simulink model "LATC_Test_Calc4"  (R2021b)
settings: Solver=FixedStepDiscrete  StartTime=49.3316  StopTime=94.3708  FixedStep=0.01  RelTol=1e-3
values from neighbouring files (symbols this model uses):
  P_Global_CharSpd_ms : value not decoded    [PubParsGlobal.sldd]
  P_Global_SteeringAngleRatio : value not decoded    [PubParsGlobal.sldd]
  P_Global_WheelBase_m : value not decoded    [PubParsGlobal.sldd]
  P_LCS_Current_Offset_Test_SW = 0.0    [LATC.sldd]
  P_LCS_Current_Offset_Test_Value = 0.0    [LATC.sldd]
  P_LCS_Curvature_bp : value not decoded    [LATC.sldd]
  P_LCS_CycleTime = 0.4 0.4 0.4 0.4 0.4 0.4 0.4 0.4 0.4 0.6 0.6 0.6 0.6 0.6 0.6 0.6 0.4 0.4 0.4 0.4 0.4 0.4 0.4 0.4 0.4 0.6 0.6 0.6 0.6 0.6 0.6 0.6 0.4 0.4 0.4 0.4 0.4 0.4 0.4 0.4 0.4 0.6 0.6 0.6 0.6 0.6 0.6 0.6 0.4 0.4 0.4 0.4 0.4 0.4 0.4 0.4 0.4 0.6 0.6 0.6 0.6 0.6 0.6 0.6 0.4 0.4 0.4 0.4 0.4 0.4 0.4 0.4 0.4 0.6 0.6 0.6 0.6 0.6 0.6 0.6 0.4 0.4 0.4 0.4 0.4 0.4 0.4 0.4 0.4 0.6 0.6 0.6 0.6 0.6 0.6 0.6 0.4 0.4 0.4 0.4    [LATC.sldd]
  P_LCS_ESS_AngleSlope_Limit = 2.9    [LATC.sldd]    (also in LCS_v05.sldd)
  P_LCS_LATC_CurOffsetVehicleSpdLimitValue_degs = 7.0    [LATC.sldd]
  P_LCS_LATC_Du_Max = 20.0    [LATC.sldd]
  P_LCS_LATC_ELKAngleSlope_ratio : value not decoded    [LATC.sldd]
  P_LCS_LATC_ELKMaxLatAcc_ms2 : value not decoded    [LATC.sldd]
  P_LCS_LATC_ESSAngleSlope_ratio : value not decoded    [LATC.sldd]
  P_LCS_LATC_ESSMaxLatAcc_ms2 : value not decoded    [LATC.sldd]
  P_LCS_LATC_LCAngleSlope_ratio : value not decoded    [LATC.sldd]
  P_LCS_LATC_LCCancleMaxLatAcc_ms2 : value not decoded    [LATC.sldd]
  P_LCS_LATC_LCEcoAngleSlope_ratio : value not decoded    [LATC.sldd]
  P_LCS_LATC_LCEcoMaxLatAcc_ms2 : value not decoded    [LATC.sldd]
  P_LCS_LATC_LCKAngleSlope_ratio : value not decoded    [LATC.sldd]
  P_LCS_LATC_LCKIEAngleSlope_ratio : value not decoded    [LATC.sldd]
  P_LCS_LATC_LCKIEMaxLatAcc_ms2 : value not decoded    [LATC.sldd]
  P_LCS_LATC_LCKMaxLatAcc_ms2 : value not decoded    [LATC.sldd]
  P_LCS_LATC_LCNormalAngleSlope_ratio : value not decoded    [LATC.sldd]
  P_LCS_LATC_LCNormalMaxLatAcc_ms2 : value not decoded    [LATC.sldd]
  P_LCS_LATC_LCSportAngleSlope_ratio : value not decoded    [LATC.sldd]
  P_LCS_LATC_LCSportMaxLatAcc_ms2 : value not decoded    [LATC.sldd]
  P_LCS_LATC_LKAAngleSlope_ratio : value not decoded    [LATC.sldd]
  P_LCS_LATC_LKAMaxLatAcc_ms2 : value not decoded    [LATC.sldd]
  P_LCS_LATC_MatrixQ1_st = 0.8 0.8 1.2 1.4 1.4 1.4 2.0 2.2 2.2 2.2 2.2 2.2 2.2 2.2 2.2 2.2 0.8 0.8 1.2 1.4 1.4 1.4 2.0 2.2 2.2 2.2 2.2 2.2 2.2 2.2 2.2 2.2 0.8 0.8 1.2 1.4 1.4 1.4 2.0 2.2 2.2 2.2 2.2 2.2 2.2 2.2 2.2 2.2 0.8 0.8 1.2 1.4 1.4 1.4 2.0 2.2 2.2 2.2 2.2 2.2 2.2 2.2 2.2 2.2 0.8 0.8 1.2 1.4 1.4 1.4 2.0 2.2 2.2 2.2 2.2 2.2 2.2 2.2 2.2 2.2 0.8 0.8 1.2 1.4 1.4 1.4 2.0 2.2 2.2 2.2 2.2 2.2 2.2 2.2 2.2 2.2 0.8 0.8 1.2 1.4    [LATC.sldd]
  P_LCS_LATC_MatrixQ3_st = 20.0 20.0 20.0 20.0 20.0 15.0 15.0 15.0 15.0 15.0 15.0 15.0 15.0 13.0 13.0 13.0 20.0 20.0 20.0 20.0 20.0 15.0 15.0 15.0 15.0 15.0 15.0 15.0 15.0 13.0 13.0 13.0 20.0 20.0 20.0 20.0 20.0 15.0 15.0 15.0 15.0 15.0 15.0 15.0 15.0 13.0 13.0 13.0 20.0 20.0 20.0 20.0 20.0 15.0 15.0 15.0 15.0 15.0 15.0 15.0 15.0 13.0 13.0 13.0 20.0 20.0 20.0 20.0 20.0 15.0 15.0 15.0 15.0 15.0 15.0 15.0 15.0 13.0 13.0 13.0    [LATC.sldd]
  P_LCS_LATC_MatrixR_st = 10.0 10.0 10.0 10.0 10.0 10.0 10.0 15.0 15.0 15.0 15.0 15.0 15.0 15.0 15.0 15.0 10.0 10.0 10.0 10.0 10.0 10.0 10.0 15.0 15.0 15.0 15.0 15.0 15.0 15.0 15.0 15.0 10.0 10.0 10.0 10.0 10.0 10.0 10.0 15.0 15.0 15.0 15.0 15.0 15.0 15.0 15.0 15.0 10.0 10.0 10.0 10.0 10.0 10.0 10.0 15.0 15.0 15.0 15.0 15.0 15.0 15.0 15.0 15.0 10.0 10.0 10.0 10.0 10.0 10.0 10.0 15.0 15.0 15.0 15.0 15.0 15.0 15.0 15.0 15.0    [LATC.sldd]
  P_LCS_LATC_Max_LatAcc = 4.0    [LATC.sldd]
  P_LCS_LATC_Max_Phi = 15.0    [LATC.sldd]
  P_LCS_LATC_Max_y = 0.5    [LATC.sldd]
  P_LCS_LATC_MPC_SW = 0.0    [LATC.sldd]
  P_LCS_LATC_PreView_SW = 1.0    [LATC.sldd]
  P_LCS_LATC_SoftConstWeight = 1.0    [LATC.sldd]
  P_LCS_LATC_StateActivAngleSlopeLimit_ratio : value not decoded    [LATC.sldd]
  P_LCS_LATC_StateActiveFlg_TabX_st : value not decoded    [LATC.sldd]
  P_LCS_LATC_StateActiveHoldTime_TabY_st : value not decoded    [LATC.sldd]
  P_LCS_LATC_StateHoldTime_st = 250.0    [LATC.sldd]
  P_LCS_LATC_TarAngleFliterWindowSize = 5.0    [LATC.sldd]
  P_LCS_LATC_TarAngleLP_Time = 0.02    [LATC.sldd]
  P_LCS_LATC_U_Max = 90.0    [LATC.sldd]
  P_LCS_LCK_AngleSlope_Limit = 1.4    [LATC.sldd]
  P_LCS_LineVaildSW = 0.0    [LATC.sldd]
  P_LCS_Lookahead_Distance : value not decoded    [LATC.sldd]
  P_LCS_Lookahead_DistanceFac : value not decoded    [LATC.sldd]
  P_LCS_PLAN_CurvePreView_s = 0.3    [LATC.sldd]
  P_LCS_PLAN_CurvePreview_TabX_m : value not decoded    [LATC.sldd]
  P_LCS_PLAN_CurvePreViewFilterTime_s = 0.1    [LATC.sldd]
  P_LCS_PLAN_ELKAyDtLimit_Tab_ms3 = 1.0 1.0 1.0 1.0 1.0 1.0 1.0 1.0 1.0 1.0 1.0 1.0 1.0 1.0 1.0 1.0 1.0 1.0 1.0 1.0 1.0 1.0 1.0 1.0 1.0 1.0 1.0 1.0 1.0 1.0 1.0 1.0 1.0 1.0 1.0 1.0 1.0 1.0 1.0 1.0 1.0 1.0 1.0 1.0 1.0 1.0 1.0 1.0 1.0 1.0 1.0 1.0 1.0 1.0 1.0 1.0 1.0 1.0 1.0 1.0 1.0 1.0 1.0 1.0 1.0 1.0 1.0 1.0 1.0 1.0 1.0 1.0 1.0 1.0 1.0 1.0 1.0 1.0 1.0 1.0 1.0 1.0 1.0 1.0 1.0 1.0 1.0 1.0 1.0 1.0 1.0 1.0 1.0 1.0 1.0 1.0 1.0 1.0 1.0 1.0    [LATC.sldd]
  P_LCS_PLAN_ESSAyDtLimit_Tab_ms3 = 1.0 1.0 1.0 1.0 1.0 1.0 1.0 1.0 1.0 1.0 1.0 1.0 1.0 1.0 1.0 1.0 1.0 1.0 1.0 1.0 1.0 1.0 1.0 1.0 1.0 1.0 1.0 1.0 1.0 1.0 1.0 1.0 1.0 1.0 1.0 1.0 1.0 1.0 1.0 1.0 1.0 1.0 1.0 1.0 1.0 1.0 1.0 1.0 1.0 1.0 1.0 1.0 1.0 1.0 1.0 1.0 1.0 1.0 1.0 1.0 1.0 1.0 1.0 1.0 1.0 1.0 1.0 1.0 1.0 1.0 1.0 1.0 1.0 1.0 1.0 1.0 1.0 1.0 1.0 1.0 1.0 1.0 1.0 1.0 1.0 1.0 1.0 1.0 1.0 1.0 1.0 1.0 1.0 1.0 1.0 1.0 1.0 1.0 1.0 1.0    [LATC.sldd]
  P_LCS_PLAN_LCCancleAyDtLimit_Tab_ms3 = 1.0 1.0 1.0 1.0 1.0 1.0 1.0 1.0 1.0 1.0 1.0 1.0 1.0 1.0 1.0 1.0 1.0 1.0 1.0 1.0 1.0 1.0 1.0 1.0 1.0 1.0 1.0 1.0 1.0 1.0 1.0 1.0 1.0 1.0 1.0 1.0 1.0 1.0 1.0 1.0 1.0 1.0 1.0 1.0 1.0 1.0 1.0 1.0 1.0 1.0 1.0 1.0 1.0 1.0 1.0 1.0 1.0 1.0 1.0 1.0 1.0 1.0 1.0 1.0 1.0 1.0 1.0 1.0 1.0 1.0 1.0 1.0 1.0 1.0 1.0 1.0 1.0 1.0 1.0 1.0 1.0 1.0 1.0 1.0 1.0 1.0 1.0 1.0 1.0 1.0 1.0 1.0 1.0 1.0 1.0 1.0 1.0 1.0 1.0 1.0    [LATC.sldd]
  P_LCS_PLAN_LCEcoAyDtLimit_Tab_ms3 = 1.0 1.0 1.0 1.0 1.0 1.0 1.0 1.0 1.0 1.0 1.0 1.0 1.0 1.0 1.0 1.0 1.0 1.0 1.0 1.0 1.0 1.0 1.0 1.0 1.0 1.0 1.0 1.0 1.0 1.0 1.0 1.0 1.0 1.0 1.0 1.0 1.0 1.0 1.0 1.0 1.0 1.0 1.0 1.0 1.0 1.0 1.0 1.0 1.0 1.0 1.0 1.0 1.0 1.0 1.0 1.0 1.0 1.0 1.0 1.0 1.0 1.0 1.0 1.0 1.0 1.0 1.0 1.0 1.0 1.0 1.0 1.0 1.0 1.0 1.0 1.0 1.0 1.0 1.0 1.0 1.0 1.0 1.0 1.0 1.0 1.0 1.0 1.0 1.0 1.0 1.0 1.0 1.0 1.0 1.0 1.0 1.0 1.0 1.0 1.0    [LATC.sldd]
  P_LCS_PLAN_LCKAyDtLimit_Tab_ms3 = 1.5 1.5 1.5 1.5 1.5 1.5 1.5 1.5 1.5 1.5 1.5 1.5 1.5 1.5 1.5 1.5 1.5 1.5 1.5 1.5 1.5 1.5 1.5 1.5 1.5 1.5 1.5 1.5 1.5 1.5 1.5 1.5 1.5 1.5 1.5 1.5 1.5 1.5 1.5 1.5 1.5 1.5 1.5 1.5 1.5 1.5 1.5 1.5 1.5 1.5 1.5 1.5 1.5 1.5 1.5 1.5 1.5 1.5 1.5 1.5 1.5 1.5 1.5 1.5 1.5 1.5 1.5 1.5 1.5 1.5 1.5 1.5 1.5 1.5 1.5 1.5 1.5 1.5 1.5 1.5 1.5 1.5 1.5 1.5 1.5 1.5 1.5 1.5 1.5 1.5 1.5 1.5 1.5 1.5 1.5 1.5 1.5 1.5 1.5 1.5    [LATC.sldd]
  P_LCS_PLAN_LCKIEAyDtLimit_Tab_ms3 = 1.0 1.0 1.0 1.0 1.0 1.0 1.0 1.0 1.0 1.0 1.0 1.0 1.0 1.0 1.0 1.0 1.0 1.0 1.0 1.0 1.0 1.0 1.0 1.0 1.0 1.0 1.0 1.0 1.0 1.0 1.0 1.0 1.0 1.0 1.0 1.0 1.0 1.0 1.0 1.0 1.0 1.0 1.0 1.0 1.0 1.0 1.0 1.0 1.0 1.0 1.0 1.0 1.0 1.0 1.0 1.0 1.0 1.0 1.0 1.0 1.0 1.0 1.0 1.0 1.0 1.0 1.0 1.0 1.0 1.0 1.0 1.0 1.0 1.0 1.0 1.0 1.0 1.0 1.0 1.0 1.0 1.0 1.0 1.0 1.0 1.0 1.0 1.0 1.0 1.0 1.0 1.0 1.0 1.0 1.0 1.0 1.0 1.0 1.0 1.0    [LATC.sldd]
  P_LCS_PLAN_LCNormalAyDtLimit_Tab_ms3 = 1.0 1.0 1.0 1.0 1.0 1.0 1.0 1.0 1.0 1.0 1.0 1.0 1.0 1.0 1.0 1.0 1.0 1.0 1.0 1.0 1.0 1.0 1.0 1.0 1.0 1.0 1.0 1.0 1.0 1.0 1.0 1.0 1.0 1.0 1.0 1.0 1.0 1.0 1.0 1.0 1.0 1.0 1.0 1.0 1.0 1.0 1.0 1.0 1.0 1.0 1.0 1.0 1.0 1.0 1.0 1.0 1.0 1.0 1.0 1.0 1.0 1.0 1.0 1.0 1.0 1.0 1.0 1.0 1.0 1.0 1.0 1.0 1.0 1.0 1.0 1.0 1.0 1.0 1.0 1.0 1.0 1.0 1.0 1.0 1.0 1.0 1.0 1.0 1.0 1.0 1.0 1.0 1.0 1.0 1.0 1.0 1.0 1.0 1.0 1.0    [LATC.sldd]
  P_LCS_PLAN_LCSportAyDtLimit_Tab_ms3 = 1.0 1.0 1.0 1.0 1.0 1.0 1.0 1.0 1.0 1.0 1.0 1.0 1.0 1.0 1.0 1.0 1.0 1.0 1.0 1.0 1.0 1.0 1.0 1.0 1.0 1.0 1.0 1.0 1.0 1.0 1.0 1.0 1.0 1.0 1.0 1.0 1.0 1.0 1.0 1.0 1.0 1.0 1.0 1.0 1.0 1.0 1.0 1.0 1.0 1.0 1.0 1.0 1.0 1.0 1.0 1.0 1.0 1.0 1.0 1.0 1.0 1.0 1.0 1.0 1.0 1.0 1.0 1.0 1.0 1.0 1.0 1.0 1.0 1.0 1.0 1.0 1.0 1.0 1.0 1.0 1.0 1.0 1.0 1.0 1.0 1.0 1.0 1.0 1.0 1.0 1.0 1.0 1.0 1.0 1.0 1.0 1.0 1.0 1.0 1.0    [LATC.sldd]
  P_LCS_PLAN_LKAAyDtLimit_Tab_ms3 = 1.0 1.0 1.0 1.0 1.0 1.0 1.0 1.0 1.0 1.0 1.0 1.0 1.0 1.0 1.0 1.0 1.0 1.0 1.0 1.0 1.0 1.0 1.0 1.0 1.0 1.0 1.0 1.0 1.0 1.0 1.0 1.0 1.0 1.0 1.0 1.0 1.0 1.0 1.0 1.0 1.0 1.0 1.0 1.0 1.0 1.0 1.0 1.0 1.0 1.0 1.0 1.0 1.0 1.0 1.0 1.0 1.0 1.0 1.0 1.0 1.0 1.0 1.0 1.0 1.0 1.0 1.0 1.0 1.0 1.0 1.0 1.0 1.0 1.0 1.0 1.0 1.0 1.0 1.0 1.0 1.0 1.0 1.0 1.0 1.0 1.0 1.0 1.0 1.0 1.0 1.0 1.0 1.0 1.0 1.0 1.0 1.0 1.0 1.0 1.0    [LATC.sldd]
  P_LCS_PLAN_MinPlanDis_m : value not decoded    [LATC.sldd]
  P_LCS_PLAN_PreCurMinDisFac_ratio : value not decoded    [LATC.sldd]
  P_LCS_PLAN_PreDisCurve_TabX_m : value not decoded    [LATC.sldd]
  P_LCS_PLAN_StateActiv_AyDtLimit_ms3 : value not decoded    [LATC.sldd]
  P_LCS_PLAN_VehicleSpd_TabX_kph : value not decoded    [LATC.sldd]
  P_LCS_PLAN_VehicleSpd_TabY_Kph : value not decoded    [LATC.sldd]
  P_LCS_VehicleSpd_TabX_Kph : value not decoded    [LATC.sldd]
libraries: simulink x3, dspbuff3 x2
(part 3 of 4)

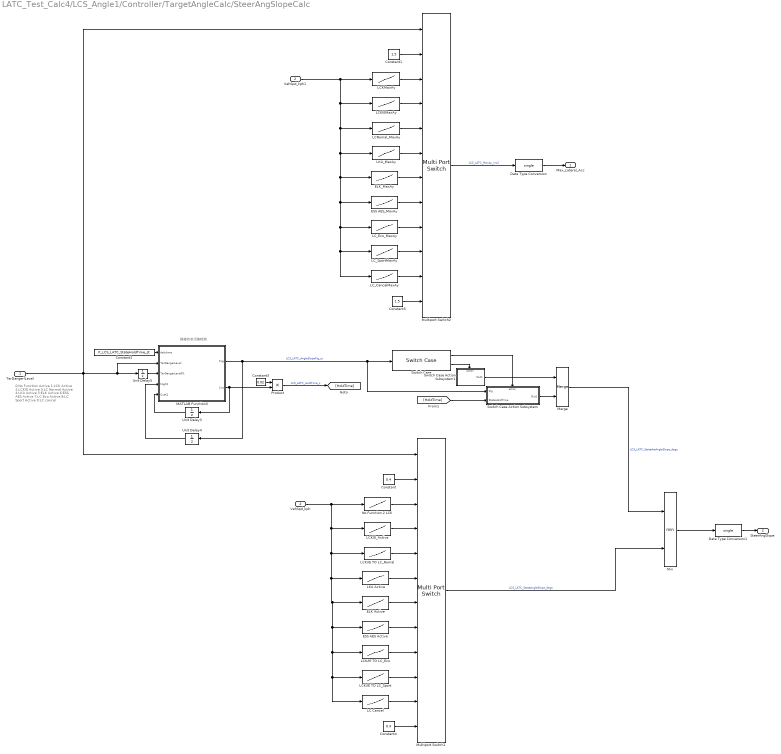
== system LATC_Test_Calc4/LCS_Angle1/Controller/TargetAngleCalc/SteerAngSlopeCalc ==
  note: 0:No Function Active
      | 1:LCK Active
      | 2:LCKIE Active
      | 3:LC Normal Active
      | 4:LKA Active
      | 5:ELK Active
      | 6:ESS AES Active
      | 7:LC Eco Active
      | 8:LC Sport Active
      | 9:LC cancel
  note: 换道状态切换检测
  TarDangerlLevel : Inport
  VehSpd_kph : Inport  Port=2
  Constant : Constant  Value=0.4  OutDataTypeStr=single
  Constant1 : Constant  Value=1.5  OutDataTypeStr=single
  Constant2 : Constant  Value=P_LCS_LATC_StateHoldTime_st  OutDataTypeStr=uint16
  Constant3 : Constant  Value=0.02
  Constant4 : Constant  Value=0.4  OutDataTypeStr=single
  Constant5 : Constant  Value=1.5  OutDataTypeStr=single
  Data Type Conversion : DataTypeConversion  OutDataTypeStr=single
  Data Type Conversion1 : DataTypeConversion  OutDataTypeStr=single
  ELK Active : Lookup_n-D  NumberOfTableDimensions=1  BreakpointsForDimension1=P_LCS_VehicleSpd_TabX_Kph  Table=P_LCS_LATC_ELKAngleSlope_ratio  ExtrapMethod=Clip  InternalRulePriority=Speed  RndMeth=Simplest  InputSameDT=on
  ELK_MaxAy : Lookup_n-D  NumberOfTableDimensions=1  BreakpointsForDimension1=P_LCS_VehicleSpd_TabX_Kph  Table=P_LCS_LATC_ELKMaxLatAcc_ms2  ExtrapMethod=Clip  InternalRulePriority=Speed  RndMeth=Simplest  InputSameDT=on
  ESS AES Active : Lookup_n-D  NumberOfTableDimensions=1  BreakpointsForDimension1=P_LCS_VehicleSpd_TabX_Kph  Table=P_LCS_LATC_ESSAngleSlope_ratio  ExtrapMethod=Clip  InternalRulePriority=Speed  RndMeth=Simplest  InputSameDT=on
  ESS AES_MaxAy : Lookup_n-D  NumberOfTableDimensions=1  BreakpointsForDimension1=P_LCS_VehicleSpd_TabX_Kph  Table=P_LCS_LATC_ESSMaxLatAcc_ms2  ExtrapMethod=Clip  InternalRulePriority=Speed  RndMeth=Simplest  InputSameDT=on
  LC Cancel : Lookup_n-D  NumberOfTableDimensions=1  BreakpointsForDimension1=P_LCS_VehicleSpd_TabX_Kph  Table=P_LCS_LATC_LCAngleSlope_ratio  ExtrapMethod=Clip  InternalRulePriority=Speed  RndMeth=Simplest  InputSameDT=on
  LCK/IE TO LC_Eco : Lookup_n-D  NumberOfTableDimensions=1  BreakpointsForDimension1=P_LCS_VehicleSpd_TabX_Kph  Table=P_LCS_LATC_LCEcoAngleSlope_ratio  ExtrapMethod=Clip  InternalRulePriority=Speed  RndMeth=Simplest  InputSameDT=on
  LCK/IE TO LC_Nomal : Lookup_n-D  NumberOfTableDimensions=1  BreakpointsForDimension1=P_LCS_VehicleSpd_TabX_Kph  Table=P_LCS_LATC_LCNormalAngleSlope_ratio  ExtrapMethod=Clip  InternalRulePriority=Speed  RndMeth=Simplest  InputSameDT=on
  LCK/IE TO LC_Sport : Lookup_n-D  NumberOfTableDimensions=1  BreakpointsForDimension1=P_LCS_VehicleSpd_TabX_Kph  Table=P_LCS_LATC_LCSportAngleSlope_ratio  ExtrapMethod=Clip  InternalRulePriority=Speed  RndMeth=Simplest  InputSameDT=on
  LCKIEMaxAy : Lookup_n-D  NumberOfTableDimensions=1  BreakpointsForDimension1=P_LCS_VehicleSpd_TabX_Kph  Table=P_LCS_LATC_LCKIEMaxLatAcc_ms2  ExtrapMethod=Clip  InternalRulePriority=Speed  RndMeth=Simplest  InputSameDT=on
  LCKIE_Active : Lookup_n-D  NumberOfTableDimensions=1  BreakpointsForDimension1=P_LCS_VehicleSpd_TabX_Kph  Table=P_LCS_LATC_LCKIEAngleSlope_ratio  ExtrapMethod=Clip  InternalRulePriority=Speed  RndMeth=Simplest  InputSameDT=on
  LCKMaxAy : Lookup_n-D  NumberOfTableDimensions=1  BreakpointsForDimension1=P_LCS_VehicleSpd_TabX_Kph  Table=P_LCS_LATC_LCKMaxLatAcc_ms2  ExtrapMethod=Clip  InternalRulePriority=Speed  RndMeth=Simplest  InputSameDT=on
  LCNomal_MaxAy : Lookup_n-D  NumberOfTableDimensions=1  BreakpointsForDimension1=P_LCS_VehicleSpd_TabX_Kph  Table=P_LCS_LATC_LCNormalMaxLatAcc_ms2  ExtrapMethod=Clip  InternalRulePriority=Speed  RndMeth=Simplest  InputSameDT=on
  LC_CancelMaxAy : Lookup_n-D  NumberOfTableDimensions=1  BreakpointsForDimension1=P_LCS_VehicleSpd_TabX_Kph  Table=P_LCS_LATC_LCCancleMaxLatAcc_ms2  ExtrapMethod=Clip  InternalRulePriority=Speed  RndMeth=Simplest  InputSameDT=on
  LC_Eco_MaxAy : Lookup_n-D  NumberOfTableDimensions=1  BreakpointsForDimension1=P_LCS_VehicleSpd_TabX_Kph  Table=P_LCS_LATC_LCEcoMaxLatAcc_ms2  ExtrapMethod=Clip  InternalRulePriority=Speed  RndMeth=Simplest  InputSameDT=on
  LC_SportMaxAy : Lookup_n-D  NumberOfTableDimensions=1  BreakpointsForDimension1=P_LCS_VehicleSpd_TabX_Kph  Table=P_LCS_LATC_LCSportMaxLatAcc_ms2  ExtrapMethod=Clip  InternalRulePriority=Speed  RndMeth=Simplest  InputSameDT=on
  LKA Active : Lookup_n-D  NumberOfTableDimensions=1  BreakpointsForDimension1=P_LCS_VehicleSpd_TabX_Kph  Table=P_LCS_LATC_LKAAngleSlope_ratio  ExtrapMethod=Clip  InternalRulePriority=Speed  RndMeth=Simplest  InputSameDT=on
  LKA_MaxAy : Lookup_n-D  NumberOfTableDimensions=1  BreakpointsForDimension1=P_LCS_VehicleSpd_TabX_Kph  Table=P_LCS_LATC_LKAMaxLatAcc_ms2  ExtrapMethod=Clip  InternalRulePriority=Speed  RndMeth=Simplest  InputSameDT=on
  MATLAB Function3 : MATLAB Function  TreatAsAtomicUnit=on
  Merge : Merge
  Min : MinMax  Inputs=2
  Multiport Switch1 : MultiPortSwitch  DataPortOrder=Zero-based contiguous  Inputs=11  zeroidx=on
  Multiport Switch2 : MultiPortSwitch  DataPortOrder=Zero-based contiguous  Inputs=11  zeroidx=on
  No Function 2 LCK : Lookup_n-D  NumberOfTableDimensions=1  BreakpointsForDimension1=P_LCS_VehicleSpd_TabX_Kph  Table=P_LCS_LATC_LCKAngleSlope_ratio  ExtrapMethod=Clip  InternalRulePriority=Speed  RndMeth=Simplest  InputSameDT=on
  Product : Product
  Switch Case : SwitchCase  CaseConditions={[1,2,3,4,5]}
  Switch Case Action Subsystem : Subsystem  TreatAsAtomicUnit=on
  Switch Case Action Subsystem1 : Subsystem  TreatAsAtomicUnit=on
  Unit Delay3 : UnitDelay  SampleTime=-1  HasFrameUpgradeWarning=on
  Unit Delay4 : UnitDelay  SampleTime=-1  HasFrameUpgradeWarning=on
  Unit Delay5 : UnitDelay  SampleTime=-1  HasFrameUpgradeWarning=on
  VehSpd_kph1 : InportShadow  Port=2
  Max_Lateral_Acc : Outport  OutDataTypeStr=single
  SteerAngSlope : Outport  Port=2  OutDataTypeStr=single
  wires:
  TarDangerlLevel/1 -> Multiport Switch1/1, Multiport Switch2/1, Unit Delay5/1, MATLAB Function3/2(TarDangerLevel)
  Merge/1 -> Min/1  "LCS_LATC_StateActAngleSlope_degs"
  Switch Case Action Subsystem1/1(Out1) -> Merge/1
  Switch Case Action Subsystem/1(Out1) -> Merge/2
  [HoldTime] -> Switch Case Action Subsystem/2(StateHoldTime)
  Switch Case/2 -> Switch Case Action Subsystem1/Action
  Switch Case/1 -> Switch Case Action Subsystem/Action
  LCK/IE TO LC_Nomal/1 -> Multiport Switch1/5
  Min/1 -> Data Type Conversion1/1
  Product/1 -> [HoldTime]  "LCS_LATC_HoldTime_s"
  Constant3/1 -> Product/1
  Constant4/1 -> Multiport Switch1/12
  LKA Active/1 -> Multiport Switch1/6
  No Function 2 LCK/1 -> Multiport Switch1/3
  Multiport Switch1/1 -> Min/2  "LCS_LATC_StateAngleSlope_degs"
  Constant2/1 -> MATLAB Function3/1(delytime)
  MATLAB Function3/1(FLg) -> Unit Delay4/1, Switch Case Action Subsystem/1(Flg), Switch Case/1  "LCS_LATC_AngleSlopeFlg_st"
  MATLAB Function3/2(Cnt) -> Unit Delay3/1, Product/2
  Constant/1 -> Multiport Switch1/2
  Unit Delay4/1 -> MATLAB Function3/4(FLgK1)
  Unit Delay3/1 -> MATLAB Function3/5(CntK1)
  LCKIE_Active/1 -> Multiport Switch1/4
  ELK Active/1 -> Multiport Switch1/7
  VehSpd_kph/1 -> No Function 2 LCK/1, LCK/IE TO LC_Nomal/1, LC Cancel/1, LCK/IE TO LC_Sport/1, LCK/IE TO LC_Eco/1, ESS AES Active/1, ELK Active/1, LKA Active/1, LCKIE_Active/1
  Unit Delay5/1 -> MATLAB Function3/3(TarDangerLevelK1)
  ESS AES Active/1 -> Multiport Switch1/8
  LCK/IE TO LC_Eco/1 -> Multiport Switch1/9
  LCK/IE TO LC_Sport/1 -> Multiport Switch1/10
  LC Cancel/1 -> Multiport Switch1/11
  Multiport Switch2/1 -> Data Type Conversion/1  "LCS_LATC_MaxAy_ms2"
  Constant1/1 -> Multiport Switch2/2
  Constant5/1 -> Multiport Switch2/12
  LC_CancelMaxAy/1 -> Multiport Switch2/11
  LC_SportMaxAy/1 -> Multiport Switch2/10
  LC_Eco_MaxAy/1 -> Multiport Switch2/9
  ESS AES_MaxAy/1 -> Multiport Switch2/8
  VehSpd_kph1/1 -> LCKIEMaxAy/1, LKA_MaxAy/1, ELK_MaxAy/1, ESS AES_MaxAy/1, LC_Eco_MaxAy/1, LC_SportMaxAy/1, LC_CancelMaxAy/1, LCNomal_MaxAy/1, LCKMaxAy/1
  ELK_MaxAy/1 -> Multiport Switch2/7
  LCKIEMaxAy/1 -> Multiport Switch2/4
  LCKMaxAy/1 -> Multiport Switch2/3
  LKA_MaxAy/1 -> Multiport Switch2/6
  LCNomal_MaxAy/1 -> Multiport Switch2/5
  Data Type Conversion/1 -> Max_Lateral_Acc/1
  Data Type Conversion1/1 -> SteerAngSlope/1

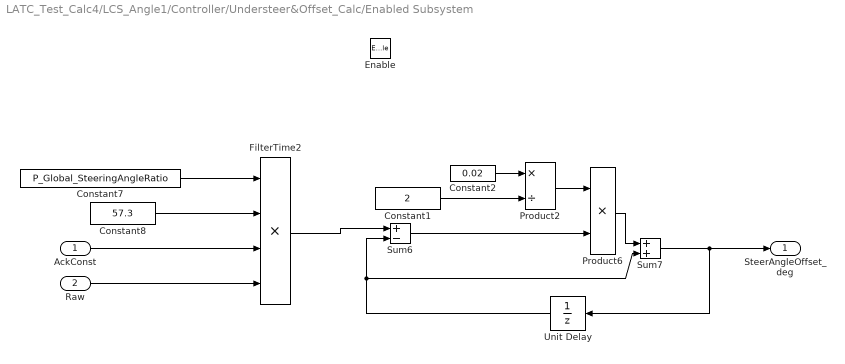
== system LATC_Test_Calc4/LCS_Angle1/Controller/Understeer&Offset_Calc/Enabled Subsystem ==
  AckConst : Inport
  Raw : Inport  Port=2
  Enable : EnablePort
  Constant1 : Constant  Value=2  OutDataTypeStr=single
  Constant2 : Constant  Value=0.02  OutDataTypeStr=single
  Constant7 : Constant  Value=P_Global_SteeringAngleRatio
  Constant8 : Constant  Value=57.3  OutDataTypeStr=single
  FilterTime2 : Product  Inputs=4  RndMeth=Zero
  Product2 : Product  Inputs=*/  RndMeth=Zero
  Product6 : Product  RndMeth=Zero
  Sum6 : Sum  Inputs=+-
  Sum7 : Sum
  Unit Delay : UnitDelay  SampleTime=-1  HasFrameUpgradeWarning=on
  SteerAngleOffset_deg : Outport
  wires:
  Constant1/1 -> Product2/2
  FilterTime2/1 -> Sum6/1
  Raw/1 -> FilterTime2/4
  AckConst/1 -> FilterTime2/3
  Constant8/1 -> FilterTime2/2
  Constant7/1 -> FilterTime2/1
  Product6/1 -> Sum7/1
  Product2/1 -> Product6/1
  Sum6/1 -> Product6/2
  Constant2/1 -> Product2/1
  Unit Delay/1 -> Sum7/2, Sum6/2
  Sum7/1 -> Unit Delay/1, SteerAngleOffset_deg/1

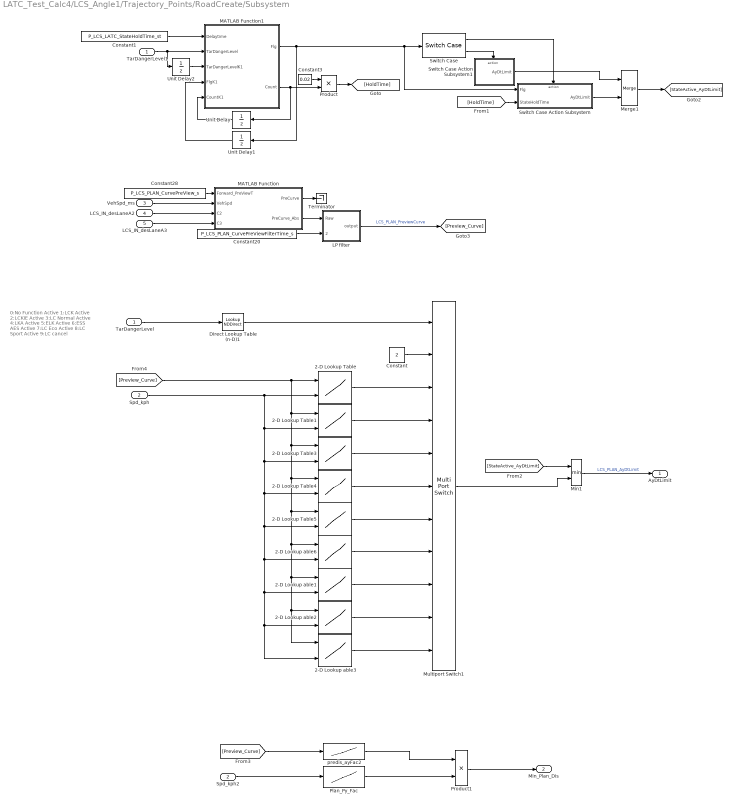
== system LATC_Test_Calc4/LCS_Angle1/Trajectory_Points/RoadCreate/Subsystem ==
  note: 0:No Function Active
      | 1:LCK Active
      | 2:LCKIE Active
      | 3:LC Normal Active
      | 4:LKA Active
      | 5:ELK Active
      | 6:ESS AES Active
      | 7:LC Eco Active
      | 8:LC Sport Active
      | 9:LC cancel
  TarDangerLevel : Inport
  Spd_kph : Inport  Port=2
  VehSpd_ms : Inport  Port=3
  LCS_IN_desLaneA2 : Inport  Port=4
  LCS_IN_desLaneA3 : Inport  Port=5
  2-D Lookup Table : Lookup_n-D  BreakpointsForDimension1=P_LCS_PLAN_PreDisCurve_TabX_m  BreakpointsForDimension2=P_LCS_PLAN_VehicleSpd_TabY_Kph  Table=P_LCS_PLAN_LCKAyDtLimit_Tab_ms3  InternalRulePriority=Speed  RndMeth=Simplest  InputSameDT=on
      settings: InputPortMap=u0,u1
  2-D Lookup Table1 : Lookup_n-D  BreakpointsForDimension1=P_LCS_PLAN_PreDisCurve_TabX_m  BreakpointsForDimension2=P_LCS_PLAN_VehicleSpd_TabY_Kph  Table=P_LCS_PLAN_LCKIEAyDtLimit_Tab_ms3  InternalRulePriority=Speed  RndMeth=Simplest  InputSameDT=on
      settings: InputPortMap=u0,u1
  2-D Lookup Table3 : Lookup_n-D  BreakpointsForDimension1=P_LCS_PLAN_PreDisCurve_TabX_m  BreakpointsForDimension2=P_LCS_PLAN_VehicleSpd_TabY_Kph  Table=P_LCS_PLAN_LCNormalAyDtLimit_Tab_ms3  InternalRulePriority=Speed  RndMeth=Simplest  InputSameDT=on
      settings: InputPortMap=u0,u1
  2-D Lookup Table4 : Lookup_n-D  BreakpointsForDimension1=P_LCS_PLAN_PreDisCurve_TabX_m  BreakpointsForDimension2=P_LCS_PLAN_VehicleSpd_TabY_Kph  Table=P_LCS_PLAN_LKAAyDtLimit_Tab_ms3  InternalRulePriority=Speed  RndMeth=Simplest  InputSameDT=on
      settings: InputPortMap=u0,u1
  2-D Lookup Table5 : Lookup_n-D  BreakpointsForDimension1=P_LCS_PLAN_PreDisCurve_TabX_m  BreakpointsForDimension2=P_LCS_PLAN_VehicleSpd_TabY_Kph  Table=P_LCS_PLAN_ELKAyDtLimit_Tab_ms3  InternalRulePriority=Speed  RndMeth=Simplest  InputSameDT=on
      settings: InputPortMap=u0,u1
  2-D Lookup able1 : Lookup_n-D  BreakpointsForDimension1=P_LCS_PLAN_PreDisCurve_TabX_m  BreakpointsForDimension2=P_LCS_PLAN_VehicleSpd_TabY_Kph  Table=P_LCS_PLAN_LCEcoAyDtLimit_Tab_ms3  InternalRulePriority=Speed  RndMeth=Simplest  InputSameDT=on
      settings: InputPortMap=u0,u1
  2-D Lookup able2 : Lookup_n-D  BreakpointsForDimension1=P_LCS_PLAN_PreDisCurve_TabX_m  BreakpointsForDimension2=P_LCS_PLAN_VehicleSpd_TabY_Kph  Table=P_LCS_PLAN_LCSportAyDtLimit_Tab_ms3  InternalRulePriority=Speed  RndMeth=Simplest  InputSameDT=on
      settings: InputPortMap=u0,u1
  2-D Lookup able3 : Lookup_n-D  BreakpointsForDimension1=P_LCS_PLAN_PreDisCurve_TabX_m  BreakpointsForDimension2=P_LCS_PLAN_VehicleSpd_TabY_Kph  Table=P_LCS_PLAN_LCCancleAyDtLimit_Tab_ms3  InternalRulePriority=Speed  RndMeth=Simplest  InputSameDT=on
      settings: InputPortMap=u0,u1
  2-D Lookup able6 : Lookup_n-D  BreakpointsForDimension1=P_LCS_PLAN_PreDisCurve_TabX_m  BreakpointsForDimension2=P_LCS_PLAN_VehicleSpd_TabY_Kph  Table=P_LCS_PLAN_ESSAyDtLimit_Tab_ms3  InternalRulePriority=Speed  RndMeth=Simplest  InputSameDT=on
      settings: InputPortMap=u0,u1
  Constant : Constant  Value=2  OutDataTypeStr=single
  Constant1 : Constant  Value=P_LCS_LATC_StateHoldTime_st  OutDataTypeStr=uint16
  Constant20 : Constant  Value=P_LCS_PLAN_CurvePreViewFilterTime_s  OutDataTypeStr=single
  Constant28 : Constant  Value=P_LCS_PLAN_CurvePreView_s  OutDataTypeStr=single
  Constant3 : Constant  Value=0.02
  Direct Lookup Table (n-D)1 : LookupNDDirect  NumberOfTableDimensions=1  Table=[0 1 2 3 4 5 6 7 8 9]  TableDataTypeStr=uint8
  LP filter : Subsystem
  MATLAB Function : MATLAB Function  TreatAsAtomicUnit=on
  MATLAB Function1 : MATLAB Function  TreatAsAtomicUnit=on
  Merge1 : Merge
  Min1 : MinMax  Inputs=2
  Multiport Switch1 : MultiPortSwitch  DataPortOrder=Zero-based contiguous  Inputs=10  zeroidx=on
  Plan_Py_Fac : Lookup_n-D  NumberOfTableDimensions=1  BreakpointsForDimension1=P_LCS_PLAN_VehicleSpd_TabX_kph  Table=P_LCS_PLAN_MinPlanDis_m  ExtrapMethod=Clip  UseLastTableValue=on  InternalRulePriority=Speed  RndMeth=Simplest  InputSameDT=on
  Product : Product
  Product1 : Product
  Spd_kph2 : InportShadow  Port=2
  Switch Case : SwitchCase  CaseConditions={[1]}
  Switch Case Action Subsystem : Subsystem  TreatAsAtomicUnit=on
  Switch Case Action Subsystem1 : Subsystem  TreatAsAtomicUnit=on
  TarDangerLevel1 : InportShadow
  Terminator : Terminator
  Unit Delay : UnitDelay  SampleTime=-1  HasFrameUpgradeWarning=on
  Unit Delay1 : UnitDelay  SampleTime=-1  HasFrameUpgradeWarning=on
  Unit Delay2 : UnitDelay  SampleTime=-1  HasFrameUpgradeWarning=on
  predis_ayFac2 : Lookup_n-D  NumberOfTableDimensions=1  BreakpointsForDimension1=P_LCS_PLAN_CurvePreview_TabX_m  Table=P_LCS_PLAN_PreCurMinDisFac_ratio  ExtrapMethod=Clip  UseLastTableValue=on  InternalRulePriority=Speed  RndMeth=Simplest  InputSameDT=on
  AyDtLimit : Outport  OutDataTypeStr=single
  Min_Plan_Dis : Outport  Port=2  OutDataTypeStr=single
  wires:
  2-D Lookup Table/1 -> Multiport Switch1/3
  Multiport Switch1/1 -> Min1/2
  [StateActive_AyDtLimit] -> Min1/1
  Merge1/1 -> [StateActive_AyDtLimit]
  Switch Case Action Subsystem1/1(AyDtLimit) -> Merge1/1
  Switch Case Action Subsystem/1(AyDtLimit) -> Merge1/2
  Product/1 -> [HoldTime]
  [HoldTime] -> Switch Case Action Subsystem/2(StateHoldTime)
  Constant3/1 -> Product/1
  Switch Case/2 -> Switch Case Action Subsystem1/Action
  MATLAB Function1/2(Count) -> Unit Delay/1, Product/2
  Switch Case/1 -> Switch Case Action Subsystem/Action
  MATLAB Function1/1(Flg) -> Switch Case/1, Switch Case Action Subsystem/1(Flg), Unit Delay1/1
  Constant1/1 -> MATLAB Function1/1(Delaytime)
  Unit Delay2/1 -> MATLAB Function1/3(TarDangerLevelK1)
  TarDangerLevel1/1 -> MATLAB Function1/2(TarDangerLevel), Unit Delay2/1
  Unit Delay1/1 -> MATLAB Function1/4(FlgK1)
  Unit Delay/1 -> MATLAB Function1/5(CountK1)
  2-D Lookup Table5/1 -> Multiport Switch1/7
  2-D Lookup Table3/1 -> Multiport Switch1/5
  2-D Lookup Table1/1 -> Multiport Switch1/4
  Constant/1 -> Multiport Switch1/2
  Constant28/1 -> MATLAB Function/1(Forward_PreViewT)
  LP filter/1(output) -> [Preview_Curve]  "LCS_PLAN_PreviewCurve"
  Constant20/1 -> LP filter/2(TorqFilterTime)
  LCS_IN_desLaneA3/1 -> MATLAB Function/4(C3)
  LCS_IN_desLaneA2/1 -> MATLAB Function/3(C2)
  VehSpd_ms/1 -> MATLAB Function/2(VehSpd)
  Min1/1 -> AyDtLimit/1  "LCS_PLAN_AyDtLimit"
  TarDangerLevel/1 -> Direct Lookup Table (n-D)1/1
  Direct Lookup Table (n-D)1/1 -> Multiport Switch1/1
  Plan_Py_Fac/1 -> Product1/2
  Spd_kph2/1 -> Plan_Py_Fac/1
  [Preview_Curve] -> predis_ayFac2/1
  Product1/1 -> Min_Plan_Dis/1
  predis_ayFac2/1 -> Product1/1
  MATLAB Function/2(PreCurve_Abs) -> LP filter/1(Raw)
  MATLAB Function/1(PreCurve) -> Terminator/1
  [Preview_Curve] -> 2-D Lookup able3/1, 2-D Lookup able2/1, 2-D Lookup able1/1, 2-D Lookup able6/1, 2-D Lookup Table5/1, 2-D Lookup Table4/1, 2-D Lookup Table3/1, 2-D Lookup Table1/1, 2-D Lookup Table/1
  Spd_kph/1 -> 2-D Lookup Table/2, 2-D Lookup Table1/2, 2-D Lookup Table3/2, 2-D Lookup Table4/2, 2-D Lookup able3/2, 2-D Lookup able2/2, 2-D Lookup able1/2, 2-D Lookup able6/2, 2-D Lookup Table5/2
  2-D Lookup Table4/1 -> Multiport Switch1/6
  2-D Lookup able6/1 -> Multiport Switch1/8
  2-D Lookup able1/1 -> Multiport Switch1/9
  2-D Lookup able2/1 -> Multiport Switch1/10
  2-D Lookup able3/1 -> Multiport Switch1/11

== system LATC_Test_Calc4/LCS_Angle1/Controller/TargetAngleCalc/MedianLowPass_Filter/LP ==
  Raw : Inport
  Constant1 : Constant  Value=P_LCS_LATC_TarAngleLP_Time  OutDataTypeStr=single
  Constant3 : Constant  Value=0.02  OutDataTypeStr=single
  Product7 : Product  Inputs=*/  RndMeth=Zero
  Product8 : Product  RndMeth=Zero
  Sum14 : Sum
  Sum9 : Sum  Inputs=+-
  Unit Delay : UnitDelay  SampleTime=-1  HasFrameUpgradeWarning=on
  Out : Outport
  wires:
  Constant1/1 -> Product7/2
  Constant3/1 -> Product7/1
  Sum9/1 -> Product8/2
  Sum14/1 -> Out/1, Unit Delay/1
  Unit Delay/1 -> Sum14/2, Sum9/2
  Raw/1 -> Sum9/1
  Product8/1 -> Sum14/1
  Product7/1 -> Product8/1

== system LATC_Test_Calc4/LCS_Angle1/Controller/TargetAngleCalc/MedianLowPass_Filter/Median_Filter ==
  In : Inport
  Add : Sum  Inputs=+-
  Constant : Constant  Value=2  OutDataTypeStr=single
  Constant11 : Constant  Value=P_LCS_LATC_TarAngleFliterWindowSize  OutDataTypeStr=single
  Delay Line : dspbuff3/Delay Line  siz=P_LCS_LATC_TarAngleFliterWindowSize  ic=0  directfeed=off  enable_output=off  hold_output=off  OutputFrames=off
      settings: SourceProductBaseCode=DS
  Divide1 : Product  Inputs=*/
  Max of Elements1 : MinMax  Function=max
  MinMax2 : MinMax
  Minus1 : Sum  Inputs=--+
  Sum of Elements1 : Sum  Inputs=+
  Out : Outport
  wires:
  Max of Elements1/1 -> Minus1/2
  Divide1/1 -> Out/1
  Minus1/1 -> Divide1/1
  In/1 -> Delay Line/1
  MinMax2/1 -> Minus1/1
  Sum of Elements1/1 -> Minus1/3
  Delay Line/1 -> Max of Elements1/1, MinMax2/1, Sum of Elements1/1
  Constant11/1 -> Add/1
  Add/1 -> Divide1/2
  Constant/1 -> Add/2

== system LATC_Test_Calc4/LCS_Angle1/Controller/TargetAngleCalc/MedianLowPass_Filter1/LP ==
  Raw : Inport
  Constant1 : Constant  Value=0.02  OutDataTypeStr=single
  Constant3 : Constant  Value=0.02  OutDataTypeStr=single
  Product7 : Product  Inputs=*/  RndMeth=Zero
  Product8 : Product  RndMeth=Zero
  Sum14 : Sum
  Sum9 : Sum  Inputs=+-
  Unit Delay : UnitDelay  SampleTime=-1  HasFrameUpgradeWarning=on
  Out : Outport
  wires:
  Constant1/1 -> Product7/2
  Constant3/1 -> Product7/1
  Sum9/1 -> Product8/2
  Sum14/1 -> Out/1, Unit Delay/1
  Unit Delay/1 -> Sum14/2, Sum9/2
  Raw/1 -> Sum9/1
  Product8/1 -> Sum14/1
  Product7/1 -> Product8/1

== system LATC_Test_Calc4/LCS_Angle1/Controller/TargetAngleCalc/MedianLowPass_Filter1/Median_Filter ==
  In : Inport
  Add : Sum  Inputs=+-
  Constant : Constant  Value=2  OutDataTypeStr=single
  Constant11 : Constant  Value=P_LCS_LATC_TarAngleFliterWindowSize  OutDataTypeStr=single
  Delay Line : dspbuff3/Delay Line  siz=P_LCS_LATC_TarAngleFliterWindowSize  ic=0  directfeed=off  enable_output=off  hold_output=off  OutputFrames=off
      settings: SourceProductBaseCode=DS
  Divide1 : Product  Inputs=*/
  Max of Elements1 : MinMax  Function=max
  MinMax2 : MinMax
  Minus1 : Sum  Inputs=--+
  Sum of Elements1 : Sum  Inputs=+
  Out : Outport
  wires:
  Max of Elements1/1 -> Minus1/2
  Divide1/1 -> Out/1
  Minus1/1 -> Divide1/1
  In/1 -> Delay Line/1
  MinMax2/1 -> Minus1/1
  Sum of Elements1/1 -> Minus1/3
  Delay Line/1 -> Max of Elements1/1, MinMax2/1, Sum of Elements1/1
  Constant11/1 -> Add/1
  Add/1 -> Divide1/2
  Constant/1 -> Add/2

== system LATC_Test_Calc4/LCS_Angle1/Controller/TargetAngleCalc/SteerAngSlopeCalc/Switch Case Action Subsystem ==
  Flg : Inport
  StateHoldTime : Inport  Port=2
  Action Port : ActionPort  ActionPortLabel=case [ 1 2 3 4 5 ]:
  LC_start_slope : Lookup_n-D  BreakpointsForDimension1=P_LCS_LATC_StateActiveFlg_TabX_st  BreakpointsForDimension2=P_LCS_LATC_StateActiveHoldTime_TabY_st  Table=P_LCS_LATC_StateActivAngleSlopeLimit_ratio  ExtrapMethod=Clip  UseLastTableValue=on  InternalRulePriority=Speed  OutDataTypeStr=single  RndMeth=Simplest
      settings: InputPortMap=u0,u1
  Out1 : Outport
  wires:
  StateHoldTime/1 -> LC_start_slope/2
  LC_start_slope/1 -> Out1/1
  Flg/1 -> LC_start_slope/1

== system LATC_Test_Calc4/LCS_Angle1/Controller/TargetAngleCalc/SteerAngSlopeCalc/Switch Case Action Subsystem1 ==
  Action Port : ActionPort  ActionPortLabel=default:
  Constant : Constant  Value=100  OutDataTypeStr=single
  Out1 : Outport
  wires:
  Constant/1 -> Out1/1

== system LATC_Test_Calc4/LCS_Angle1/Trajectory_Points/RoadCreate/Subsystem/LP filter ==
  Raw : Inport
  TorqFilterTime : Inport  Port=2
  Product1 : Product  RndMeth=Zero
  Product4 : Product  Inputs=*/  RndMeth=Zero
  Sum4 : Sum  Inputs=+-
  Sum5 : Sum
  Unit Delay : UnitDelay  SampleTime=-1  HasFrameUpgradeWarning=on
  Weight/N3 : Constant  Value=0.02  OutDataTypeStr=single
  output : Outport
  wires:
  TorqFilterTime/1 -> Product4/2
  Product4/1 -> Product1/1
  Weight/N3/1 -> Product4/1
  Raw/1 -> Sum4/1
  Product1/1 -> Sum5/1
  Sum4/1 -> Product1/2
  Unit Delay/1 -> Sum4/2, Sum5/2
  Sum5/1 -> Unit Delay/1, output/1

== system LATC_Test_Calc4/LCS_Angle1/Trajectory_Points/RoadCreate/Subsystem/Switch Case Action Subsystem ==
  Flg : Inport
  StateHoldTime : Inport  Port=2
  Action Port : ActionPort  ActionPortLabel=case [ 1 ]:
  ActiveAyDtLimit_TBL : Lookup_n-D  BreakpointsForDimension1=P_LCS_LATC_StateActiveFlg_TabX_st  BreakpointsForDimension2=P_LCS_LATC_StateActiveHoldTime_TabY_st  Table=P_LCS_PLAN_StateActiv_AyDtLimit_ms3  ExtrapMethod=Clip  UseLastTableValue=on  InternalRulePriority=Speed  OutDataTypeStr=single  RndMeth=Simplest
      settings: InputPortMap=u0,u1
  AyDtLimit : Outport
  wires:
  ActiveAyDtLimit_TBL/1 -> AyDtLimit/1
  Flg/1 -> ActiveAyDtLimit_TBL/1
  StateHoldTime/1 -> ActiveAyDtLimit_TBL/2

== system LATC_Test_Calc4/LCS_Angle1/Trajectory_Points/RoadCreate/Subsystem/Switch Case Action Subsystem1 ==
  Action Port : ActionPort  ActionPortLabel=default:
  Constant1 : Constant  Value=100  OutDataTypeStr=single
  AyDtLimit : Outport
  wires:
  Constant1/1 -> AyDtLimit/1

== matlab function LATC_Test_Calc4/LCS_Angle1/Trajectory_Points/RoadCreate/MATLAB Function4 ==
  data: C3 input; y output; C2 input; C1 input; C0 input
function y = fcn(C3,C2,C1,C0)

y = single(zeros(1,9));
y=single([C3 C2 C1 C0 0 200 1 0 0]);

end

== matlab function LATC_Test_Calc4/LCS_Angle1/Controller/StateErrorCalc/MATLAB Function ==
  data: Lookahead_Distance input; Ego_X input; Ego_Y input; Traj_X input; Traj_Y input; Traj_Heading input; Traj_Kappa input; Traj_S input; lookahead_Pt_X output; Target_Pt_X input; Target_Pt_Y input; Target_Pt_S input; lookahead_Pt_Y output; lookahead_Pt_Heading output; lookahead_Pt_Kappa output single; Lookahead_Pt_Num output
%% 为横向控制找预瞄点
function [lookahead_Pt_X,lookahead_Pt_Y,lookahead_Pt_Heading,lookahead_Pt_Kappa,Lookahead_Pt_Num]= ...
QueryLookaheadPointByPosition(Lookahead_Distance,Ego_X,Ego_Y,Traj_X,Traj_Y,Traj_Heading,Traj_Kappa,Traj_S,Target_Pt_X,Target_Pt_Y,Target_Pt_S)

    target_dist=((Target_Pt_X-Ego_X)^2+((Target_Pt_Y-Ego_Y)^2))^0.5;
    % lookahead_index=0;
    for i=1:length(Traj_X)
        %找到轨迹上累积弧长之差超过此距离的点作为预瞄点 
        %到目标点距离，再加上第i个点与目标点的弧长s之差刚好大于预瞄距离的那个点
        lookahead_dist = Traj_S(i,1)-Target_Pt_S(1,1)+target_dist;
        
        if(lookahead_dist>=Lookahead_Distance)
            lookahead_index = i;
            lookahead_Pt_X= Traj_X(lookahead_index,1);
            lookahead_Pt_Y= Traj_Y(lookahead_index,1);
            lookahead_Pt_Heading= Traj_Heading(lookahead_index,1);
            lookahead_Pt_Kappa= Traj_Kappa(lookahead_index,1);
            Lookahead_Pt_Num = i;
            return
        end
        %若遍历到最后一个点也没有大于lookahead_station的就取最后一个点
        lookahead_Pt_X= Traj_X(i,1);
        lookahead_Pt_Y= Traj_Y(i,1);
        lookahead_Pt_Heading= Traj_Heading(i,1);
        lookahead_Pt_Kappa= Traj_Kappa(i,1);
    end
    Lookahead_Pt_Num = i;
end

== matlab function LATC_Test_Calc4/LCS_Angle1/Controller/StateErrorCalc/MATLAB Function2 ==
  data: Ego_X input; Ego_Y input; Ego_Heading input; Ego_Spd input; Ego_Acc input; Ego_YawRate input; lookahead_Pt_X input; lookahead_Pt_Y input; lookahead_Pt_Heading input; lookahead_Pt_Kappa input; Project_Pt_X input; Project_Pt_Y input; Project_Pt_Heading input; Project_Pt_Kappa input; lat_error output; lat_error_rate output; heading_error output; heading_error_rate output; lat_error_lookahead output; lat_error_rate_lookahead output; heading_error_lookahead output; heading_error_rate_lookahead output
function [lat_error,lat_error_rate,heading_error,heading_error_rate,lat_error_lookahead,lat_error_rate_lookahead,heading_error_lookahead,heading_error_rate_lookahead] ...
          = ComputeLatErrors(Ego_X,Ego_Y,Ego_Heading,Ego_Spd,Ego_Acc,Ego_YawRate,lookahead_Pt_X,lookahead_Pt_Y,lookahead_Pt_Heading,lookahead_Pt_Kappa,Project_Pt_X,Project_Pt_Y,Project_Pt_Heading,Project_Pt_Kappa)
    %% 横向控制中的误差计算  
    % 感觉存在问题，打算计算两套误差状态，一个是基于车辆与垂直点的误差，一个是车辆与预瞄点的误差。再加上前边车辆的位置推算模块
    
    % 角度误差计算
    curr_heading = Ego_Heading;
    heading_error = curr_heading-Project_Pt_Heading; % 车辆朝向角与垂直点朝向角误差
    heading_error = NormalizeAngle(heading_error);
    heading_error_lookahead = curr_heading-lookahead_Pt_Heading; % 车辆朝向角与预瞄点朝向误差
    heading_error_lookahead = NormalizeAngle(heading_error_lookahead);
    % 垂直点偏差计算
    X_curr = Ego_X;
    Y_curr = Ego_Y;
    dx = X_curr - Project_Pt_X;
    dy = Y_curr - Project_Pt_Y;
    lat_error = cos(Project_Pt_Heading)*dy-sin(Project_Pt_Heading)*dx;
    lat_error_rate=Ego_Spd*sin(heading_error);
    Project_Pt_YawRate = Project_Pt_Kappa*Ego_Acc;
    heading_error_rate = Ego_YawRate-Project_Pt_YawRate;
    % 预瞄点的偏差计算
    dx_pre = X_curr - lookahead_Pt_X;
    dy_pre = Y_curr - lookahead_Pt_Y;
    lat_error_lookahead = cos(lookahead_Pt_Heading)*dy_pre-sin(lookahead_Pt_Heading)*dx_pre;
    lat_error_rate_lookahead=Ego_Spd*sin(heading_error_lookahead);
    lookahead_Pt_YawRate = lookahead_Pt_Kappa*Ego_Acc;
    heading_error_rate_lookahead = Ego_YawRate-lookahead_Pt_YawRate;
end
function res_angle=NormalizeAngle(origin_angle)
%% 角度规范化，heading角在-pi~pi之间
    res_angle=mod(origin_angle+pi,2*pi);
    if (res_angle<0)
        res_angle=res_angle+2*pi;
    end
    res_angle=res_angle-pi;
end

% tor=[cos(thetar);sin(thetar)];
% nor=[-sin(thetar);cos(thetar)];
% d_err=[x-xr;y-yr];
% ed=nor'*d_err;
% es=tor'*d_err;
% %projection_point_thetar=thetar(dmin);%apollo
% projection_point_thetar=thetar+kappar*es;
% ed_dot=vy*cos(phi-projection_point_thetar)+vx*sin(phi-projection_point_thetar);
% %%%%%%%%%
% ephi=sin(phi-projection_point_thetar);
% %%%%%%%%%
% ss_dot=vx*cos(phi-projection_point_thetar)-vy*sin(phi-projection_point_thetar);
% s_dot=ss_dot/(1-kappar*ed);
% ephi_dot=phi_dot-kappar*s_dot;

== matlab function LATC_Test_Calc4/LCS_Angle1/Controller/StateErrorCalc/Reference_Point_Select/MATLAB Function1 ==
  data: Pt1X input; Dis output; Pt1Y input; Pt2X input; Pt2Y input; AbsDis output
function [Dis,AbsDis]= fcn(Pt1X,Pt1Y,Pt2X,Pt2Y)
Dis = (sqrt((Pt1X-Pt2X)*(Pt1X-Pt2X)+(Pt1Y-Pt2Y)*(Pt1Y-Pt2Y)))*sign(Pt1Y);
AbsDis = sqrt((Pt1X-Pt2X)*(Pt1X-Pt2X)+(Pt1Y-Pt2Y)*(Pt1Y-Pt2Y));
end

== matlab function LATC_Test_Calc4/LCS_Angle1/Controller/StateErrorCalc/Reference_Point_Select/MATLAB Function2 ==
  data: path_x output; path_y output; path_x input; path_heading output; path_y input; path_kappa output; path_s output
function [path_x,path_y,path_heading,path_kappa,path_s] = fcn(path_x,path_y)
%该模块是直接采用的老王模型中的通用模块
%该函数将计算path的切线方向与x轴的夹角和曲率
%输入：path_x,y路径坐标
%输出：path heading kappa 路径的heading和曲率
%原理 heading = arctan(dy/dx);
%     kappa = dheading/ds;
%     ds = (dx^2 + dy^2)^0.5

%注意，角度的多值性会带来很大的麻烦，需要慎重处理
%例，x 与 x + 2pi往往代表同一个角度，这种多值性在计算曲率会带来麻烦
%比如 原本是(0.1 - (-0.1))/ds，但如果计算出的-0.1多了一个2pi
%kappa就等于(0.1 - (-0.1 + 2*pi))/ds，曲率会变得非常大
%还有若采用中点欧拉法计算heading时，(即使用(y2 - y1)/(x2 - x1)的反正切计算一个角度 ，用(y1 - y0)/(x1
%-x0)的反正切又计算一个角度，然后加起来除以2),如果精确值是 (a1 + a2)/2,但最终计算的结果可能是(a1 + a2 + 2pi)/2
% 还有 tan(x) = tan(x + pi) 所以arctan(tan(x))可能等于x，也可能等于x + pi
% 角度的处理非常麻烦，而且角度处理不当往往是许多奇怪错误的源头

dx = diff(path_x);
dy = diff(path_y);
%用中点欧拉法要比向前欧拉法向后欧拉法更精确，但是也可能计算出的结果比精确值多一个pi
%在这里对dx,dy做中点欧拉法，使用四象限反正切计算角度
dx_pre = [dx(1);dx];
dx_after = [dx;dx(end)];
dx_final = (dx_pre + dx_after)/2;

dy_pre = [dy(1);dy];
dy_after = [dy;dy(end)];
dy_final = (dy_pre + dy_after)/2;

ds_final = sqrt(dx_final.^2 + dy_final.^2);
cum_ds = cumsum(ds_final);
path_heading = atan2(dy_final,dx_final);

dheading = diff(path_heading);
dheading_pre = [dheading(1);dheading];
dheading_after = [dheading;dheading(end)];
dheading_final = (dheading_pre + dheading_after) / 2;
%为了防止dheading出现多一个2pi的错误，假设真实的dheading较小，用sin(dheading)近似dheading
path_kappa = sin(dheading_final) ./ ds_final;
path_s = single(zeros(length(path_x),1));
path_s(2:end,1) = cum_ds(1:end-1,1);
end

== matlab function LATC_Test_Calc4/LCS_Angle1/Controller/StateErrorCalc/Reference_Point_Select/MatchPoint_ProjectPoint ==
  data: CurPosX input; CurPosY input; MatchPtX output; MatchPtY output; MatchPtTheta output; MatchPtCurve output; MatchPtS output; RefTrajX input; ProjectPtX output; ProjectPtY output; RefTrajY input; RefTrajTheta input; RefTrajCurve input; ProjectPtTheta output; ProjectPtCurve output; RefTrajS input; ProjectPtS output
function [MatchPtX,MatchPtY,MatchPtTheta,MatchPtCurve,MatchPtS,ProjectPtX,ProjectPtY,ProjectPtTheta,ProjectPtCurve,ProjectPtS] ...
           = SearchProjectPoint(CurPosX,CurPosY,RefTrajX,RefTrajY,RefTrajTheta,RefTrajCurve,RefTrajS)
PathPtNum = single(length(RefTrajX));
Index = single(0);
MinDis = single(10000);
% 声明increase_count，用于表示在遍历时distance连续增加的个数
increase_count = 0;

for i = 1:PathPtNum
    Dis = sqrt((CurPosX-RefTrajX(i,1))*(CurPosX-RefTrajX(i,1))+(CurPosY-RefTrajY(i,1))*(CurPosY-RefTrajY(i,1)));
    if (Dis < MinDis)
        MinDis = Dis;
        Index = i;
        increase_count = 0;
    else
        increase_count = increase_count + 1;
    end
    %如果distance连续增加20次就不要再遍历了，节省时间
    if increase_count > 20
        break;
    end
end
% 找到匹配点索引MatchPoint
MatchPtX = RefTrajX(Index,1);
MatchPtY = RefTrajY(Index,1);
MatchPtTheta = RefTrajTheta(Index,1);
MatchPtCurve = RefTrajCurve(Index,1);
MatchPtS = RefTrajS(Index,1);
%求解垂直点坐标ProjectPoint
if (Index == 1) %第一个点
    PointEgoX = CurPosX;
    PointEgoY = CurPosY;
    PointA_X = RefTrajX(1,1);
    PointA_Y = RefTrajY(1,1);
    PointB_X = RefTrajX(2,1);
    PointB_Y = RefTrajY(2,1);
    DotProductA = DotProduct(PointA_X,PointA_Y,PointEgoX,PointEgoY,PointB_X,PointB_Y);
    DotProductB = DotProduct(PointB_X,PointB_Y,PointEgoX,PointEgoY,PointA_X,PointA_Y);
    if(DotProductA>=0 && DotProductB>=0)
        IndexA = single(1);
        IndexB = single(2);
    else
        IndexA = single(1);
        IndexB = single(1);
    end
elseif (Index == PathPtNum)%最后一个点
    PointEgoX = CurPosX;
    PointEgoY = CurPosY;
    PointA_X = RefTrajX(PathPtNum-1,1);
    PointA_Y = RefTrajY(PathPtNum-1,1);
    PointB_X = RefTrajX(PathPtNum,1);
    PointB_Y = RefTrajY(PathPtNum,1);
    DotProductA = DotProduct(PointA_X,PointA_Y,PointEgoX,PointEgoY,PointB_X,PointB_Y);
    DotProductB = DotProduct(PointB_X,PointB_Y,PointEgoX,PointEgoY,PointA_X,PointA_Y);
    if(DotProductA>=0 && DotProductB>=0)
        IndexA = PathPtNum-1;
        IndexB = PathPtNum;
    else
        IndexA = PathPtNum;
        IndexB = PathPtNum;
    end
else
    PointEgoX = CurPosX;
    PointEgoY = CurPosY;
    PointA_X = RefTrajX(Index,1);
    PointA_Y = RefTrajY(Index,1);
    PointB_X = RefTrajX(Index+1,1);
    PointB_Y = RefTrajY(Index+1,1);
    DotProductA = DotProduct(PointA_X,PointA_Y,PointEgoX,PointEgoY,PointB_X,PointB_Y);
    DotProductB = DotProduct(PointB_X,PointB_Y,PointEgoX,PointEgoY,PointA_X,PointA_Y);
    if(DotProductA>=0 && DotProductB>=0)
        IndexA = Index;
        IndexB = Index+1;
    else
        IndexA = Index;
        IndexB = Index-1;
    end
end
% 投影点坐标求解
PointA_X = RefTrajX(IndexA,1);
PointA_Y = RefTrajY(IndexA,1);
PointB_X = RefTrajX(IndexB,1);
PointB_Y = RefTrajY(IndexB,1);
[ProjectPtX,ProjectPtY] = Pt2LineProject(PointEgoX,PointEgoY,PointA_X,PointA_Y,PointB_X,PointB_Y);
% 求解投影点的朝向角和曲率
LengthOA = CalTwoPtLength(ProjectPtX,ProjectPtY,PointA_X,PointA_Y);
LengthAB = CalTwoPtLength(PointA_X,PointA_Y,PointB_X,PointB_Y);
if ( LengthAB < 0.001)
    fWeight = single(1);
else
    fWeight = single(LengthOA/LengthAB);
end
ProjectPtTheta = RefTrajTheta(IndexA,1)*fWeight + RefTrajTheta(IndexB,1)*(1-fWeight);
ProjectPtCurve = RefTrajCurve(IndexA,1)*fWeight + RefTrajCurve(IndexB,1)*(1-fWeight);
if IndexA > IndexB
    ProjectPtS =  RefTrajS(IndexA,1) - LengthAB*fWeight;
elseif IndexA < IndexB
    ProjectPtS =  RefTrajS(IndexA,1) + LengthAB*fWeight;
else
    ProjectPtS =  RefTrajS(IndexA,1);
end
end

function DotProduct_Result = DotProduct(X1,Y1,X2,Y2,X3,Y3)
DotProduct_Result = (X2 - X1)*(X3 - X1) + (Y2 - Y1)*(Y3 - Y1);
end
function [ProjectPtX,ProjectPtY] = Pt2LineProject(X,Y,X1,Y1,X2,Y2)
%X = single(0);Y = single(0);X1 = single(0);Y1 = single(0);X2 = single(0);Y2 = single(0);
if (abs((X2-X1)*(X2-X1) + (Y2-Y1)*(Y2-Y1)) > 0.0001)
    ProjectPtX = (X*(X2-X1)*(X2-X1)+Y*(Y2-Y1)*(X2-X1)+(X1*Y2-X2*Y1)*(Y2-Y1))/((X2-X1)*(X2-X1)+(Y2-Y1)*(Y2-Y1));
    ProjectPtY = (X*(X2-X1)*(Y2-Y1)+Y*(Y2-Y1)*(Y2-Y1)+(X2*Y1-X1*Y2)*(X2-X1))/((X2-X1)*(X2-X1)+(Y2-Y1)*(Y2-Y1));
else
    ProjectPtX = X1;
    ProjectPtY = Y1;
end
end
function Length = CalTwoPtLength(X1,Y1,X2,Y2)
Length = sqrt((X1-X2)*(X1-X2) + (Y1-Y2)*(Y1-Y2));
end
